simulink model "AME556_Project_Task2_backward"  (R2024b)
settings: Solver=daessc  StartTime=0.0  StopTime=5.5  FixedStep=0.0005  MaxStep=1e-3  RelTol=1e-2
InitFcn:
  | global params;
  | 
  | % Mass and geometry
  | params.m = 0.25;
  | params.l = 0.22;
  | params.mb = 8;
  | params.a = 0.25;
  | params.b = 0.15;
  | params.g = [0; 9.81; 0];
  | 
  | % Moment of inerita
  | Il_zz = params.m * params.l^2 / 12;
  | Ib_xx = params.mb * params.a^2 / 12;
  | Ib_yy = params.mb * params.b^2 / 12;
  | Ib_zz = params.mb * (params.a^2 + params.b^2) / 12;
  | params.Ib = diag([Ib_xx Ib_yy Ib_zz]);
  | 
  | % Spatial contact force parameters
  | Kp_g = 1e5;
  | Kd_g = 1e3;
  | 
  | % Ground contact positions
  | params.P1 = [0.0197; 0.0022; 0];
  | params.P2 = [0.1838; 0.0041; 0];
  | 
  | % State variables
  | q0 = [0.1; 0.45; 0; -pi/3; pi/2; -pi/6; pi/2]; % Initial states (before landing)
  | params.p_d = [0; 0.5; 0]; % Desired positions (after standing): [x_d; y_d; z_d];
  | params.theta_d = 0; % Desired angle
values from neighbouring files (symbols this model uses):
  dt = 0.04    [AME556_Project_Task2_CMPC_Setup.m]
  N = size(x, 2)    [AME556_HW4_P2_QP.m]    (also in AME556_Project_Task2_CMPC_Setup.m = 10)
undefined symbols (not defined in the file or in its folder): lo, P1_world0, P2_world0, X, Y, Z
libraries: nesl_utility x27, sm_lib x25
(part 2 of 2)

== matlab function AME556_Project_Task2_backward/2D Biped Robot /MATLAB Function ==
  data: dq1 input; dq2 input; dq3 input; dq4 input
function jointVelocityCheck(dq1, dq2, dq3, dq4)

dq_hip = [-30 30];
dq_knee = [-15 15];

if dq1 < dq_hip(1) || dq1 > dq_hip(2)
    error('Hip Joint 1 (%.2f) exceeds velocity limit', dq1);  
elseif dq2 < dq_knee(1) || dq2 > dq_knee(2)
    error('Knee Joint 2 (%.2f) exceeds velocity limit', dq2);  
elseif dq3 < dq_hip(1) || dq3 > dq_hip(2)
    error('Hip Joint 3 (%.2f) exceeds velocity limit', dq3);  
elseif dq4 < dq_knee(1) || dq4 > dq_knee(2)
    error('Knee Joint 4 (%.2f) exceeds velocity limit', dq4);  
end

end

== matlab function AME556_Project_Task2_backward/Controller/Condensed MPC Controller ==
  data: p input; theta input; dp input; dtheta input; qs input; tau output; P1 input; P2 input; dP1 input; dP2 input; N input; dt input; t input
%% Function: Low Level Control

function tau = lowLevelControl(p, theta, dp, dtheta, qs, P1, P2, dP1, dP2, N, dt, t)

con = gaitSchedule(N, dt, t);
F = condensed_mpc_controller(p, theta, dp, dtheta, P1, P2, N, dt, t, con);
J = jacobianFcn(theta, qs);

tau = zeros(4, 1);
if con(1, 1) && con(2, 1)
    tau = -J' * F;
elseif con(1, 1) && ~con(2, 1)
    F_swing = swingLegControl(p, dp, P2, dP2, N, dt, t);
    F_new = [F(1: 2); -F_swing];
    tau = -J' * F_new;
elseif con(2, 1) && ~con(1, 1)
    F_swing = swingLegControl(p, dp, P1, dP1, N, dt, t);
    F_new = [-F_swing; F(3: 4)];
    tau = -J' * F_new;    
end

end

%% Function: Condensed MPC Controller

function F = condensed_mpc_controller(p, theta, dp, dtheta, P1, P2, N, dt, t, con)

% Parameters
mt = 8;
a = 0.25;
b = 0.15;
g = [0; 9.81; 0];
Ib_zz = mt * (a^2 + b^2) / 12;
% Ib = diag([1 1 Ib_zz]);
% wb = [0; 0; dtheta];

numStates = 7;
numCtrls = 4;
Q = diag([200 200 800 30 30 10 0]);
R = 0.0001*eye(numCtrls);

% q = [x; y; z; R1; dx; dy; dz; wbx; wby; wbz];
% X = [x; y; theta; dx; dy; dtheta; g];
X = zeros(numStates, 1);
X(1: 2) = p;
X(3) = theta;
X(4: 5) = dp;
X(6) = dtheta;
X(7) = g(2);

% Desired states
X_d = [-0.5*t; 0.45; 0; -0.5; 0; 0; g(2)];

% Reference Trajectory
X_ref = getReferenceTrajectory(dt, N, p, theta, dp, dtheta, X_d);
y = reshape(X_ref, [numStates*N 1]);

r1 = P1 - p;
r2 = P2 - p;

% Linearized system (A, B)
A = [zeros(3)   eye(3)    zeros(3,1);
     zeros(3, numStates-1) [0; -1; 0];
     zeros(1, numStates)];

B = [zeros(3, numCtrls);
     eye(2)/mt eye(2)/mt;
     -r1(2)/Ib_zz r1(1)/Ib_zz -r2(2)/Ib_zz r2(1)/Ib_zz;
     zeros(1, numCtrls)];

% Discrete-time system matrices (Ak, Bk)
Ak = A * dt + eye(size(A, 1));
Bk = B * dt;

% Aqp
Aqp = [];
for i = 1: N
    Aqp = [Aqp; mpower(Ak, i)];
end

% bqp
Bqp = repmat(zeros(size(Bk)), N, N);
for i = 0: N-1
    element = mpower(Ak, i) * Bk;
    Bqp = Bqp + kron(diag(ones(1, N - i), -i), element);
end

% Condensation
L = kron(eye(N), Q);
K = kron(eye(N), R);

% Optimization weights (H, f)
H = 2*(Bqp'*L*Bqp + K);
f = 2*Bqp'*L*(Aqp*X - y);

% Inequality constraints (A_ineq, b_ineq)
Aineq_mu = kron(eye(2), [1 -0.7; -1 -0.7]);
Aineq_mu_N = kron(eye(N), Aineq_mu);
Aineq_F = kron(eye(2), [0 1; 0 -1]);
Aineq_F_N = kron(eye(N), Aineq_F);
Aineq = [Aineq_mu_N; Aineq_F_N];

bineq_mu = repmat([0; 0; 0; 0], N, 1);
bineq_f = [];
for i = 1: N
    bineq_f = [bineq_f; [250; -10]*con(1, i); [250; -10]*con(2, i)];
end
bineq = [bineq_mu; bineq_f];

% Initial guess
u0 = zeros(length(f), 1);

% Quadratic programming
options = optimoptions('quadprog', 'Algorithm', 'active-set', 'Display', 'off');
u_mpc = quadprog(H, f, Aineq, bineq, [], [], [], [], u0, options);

% Force inputs
F = u_mpc(1: numCtrls);

end

%% Function: Get Reference Geometry

function X_ref = getReferenceTrajectory(dt, N, p, theta, dp, dtheta, X_d)

X = [p; theta; dp; dtheta; 9.81];
X_ref = repmat(X, 1, N);

for i = 1: 3
    for k = 2: N
        if X_d(i + 3) ~= 0
            X_ref(i, k) = X(i) + X_d(i+3)*((k-1)*dt);
        else
            X_ref(i, k) = X_d(i);
        end
    end
end

end

%% Function: Swing Leg Control

function F_swing = swingLegControl(p, dp, P, dP, N, dt, t)

% Leg swing height
swingHeight = 0.05;

Kp = diag([200 300]);
Kd = eye(2)*5;

ts = rem(t, N*dt/2);

% Desired leg positions
Px_d = p(1) + (1/2)*(N*dt/2)*dp(1);
Py_d = swingHeight * sin(pi*ts/(N*dt/2));

F_swing = Kp*([Px_d; Py_d] - P) + Kd*(0 - dP);

end

%% Function: Jacobian Function
% Convert contact forces to joint torques

function J = jacobianFcn(theta, qs)

l = 0.22;

q1 = qs(1); q2 = qs(2); q3 = qs(3); q4 = qs(4);

J = [l*cos(q1 + q2 + theta) + l*cos(q1 + theta), l*cos(q1 + q2 + theta),                                          0,                      0;
     l*sin(q1 + q2 + theta) + l*sin(q1 + theta), l*sin(q1 + q2 + theta),                                          0,                      0;
                                              0,                      0, l*cos(q3 + q4 + theta) + l*cos(q3 + theta), l*cos(q3 + q4 + theta);
                                              0,                      0, l*sin(q3 + q4 + theta) + l*sin(q3 + theta), l*sin(q3 + q4 + theta)];

end

%% Function: Gait Schedule
% Generate gait schedule based on walking phase

function sigma = gaitSchedule(N, dt, t)

phase = floor(t/dt);
k = rem(phase, N);

sigma_l0 = [zeros(1, N/2) ones(1, N/2)];
sigma_r0 = [ones(1, N/2) zeros(1, N/2)];

if k ~= 0
    sigma_l = [sigma_l0(k+1: N) sigma_l0(1: k)];
    sigma_r = [sigma_r0(k+1: N) sigma_r0(1: k)];
else
    sigma_l = sigma_l0;
    sigma_r = sigma_r0;
end

sigma = [sigma_l; sigma_r];

end

== matlab function AME556_Project_Task2_backward/2D Biped Robot /MATLAB Function1 ==
  data: q1_rad input; q2_rad input; q3_rad input; q4_rad input; q1_deg output; q2_deg output; q3_deg output; q4_deg output
function [q1_deg, q2_deg, q3_deg, q4_deg] = jointAngleCheck(q1_rad, q2_rad, q3_rad, q4_rad)

q_hip = [-120 30];
q_knee = [0 160];

q1_deg = rad2deg(q1_rad);
q2_deg = rad2deg(q2_rad);
q3_deg = rad2deg(q3_rad);
q4_deg = rad2deg(q4_rad);

if q1_deg < q_hip(1) || q1_deg > q_hip(2)
    error('Hip Joint 1 (%.2f) exceeds angle limit', q1_deg);  
elseif q2_deg < q_knee(1) || q2_deg > q_knee(2)
    error('Knee Joint 2 (%.2f) exceeds angle limit', q2_deg);  
elseif q3_deg < q_hip(1) || q3_deg > q_hip(2)
    error('Hip Joint 3 (%.2f) exceeds angle limit', q3_deg);  
elseif q4_deg < q_knee(1) || q4_deg > q_knee(2)
    error('Knee Joint 4 (%.2f) exceeds angle limit', q4_deg);  
end

end

== matlab function AME556_Project_Task2_backward/2D Biped Robot /MATLAB Function2 ==
  data: tau1 input; tau2 input; tau3 input; tau4 input
function jointTorqueCheck(tau1, tau2, tau3, tau4)

tau_hip = [-30 30];
tau_knee = [-60 60];

if tau1 < tau_hip(1) || tau1 > tau_hip(2)
    error('Hip Joint 1 (%.2f) exceeds torque limit', tau1);  
elseif tau2 < tau_knee(1) || tau2 > tau_knee(2)
    error('Knee Joint 2 (%.2f) exceeds torque limit', tau2);  
elseif tau3 < tau_hip(1) || tau3 > tau_hip(2)
    error('Hip Joint 3 (%.2f) exceeds torque limit', tau3);  
elseif tau4 < tau_knee(1) || tau4 > tau_knee(2)
    error('Knee Joint 4 (%.2f) exceeds torque limit', tau4);  
end

end
